simulink model "Test_07Aug2012"  (Simulink 7.7)
settings: Solver=FixedStepDiscrete  StartTime=0.0  StopTime=inf  FixedStep=0.02  RelTol=1e-3
libraries: simulink x1, utility x1
settings Model: Creator=ttcl3  LastModifiedBy=CHIEW
settings SolverCC: MaxConsecutiveMinStep=auto
settings DebuggingCC: MultiTaskRateTransMsg=warning

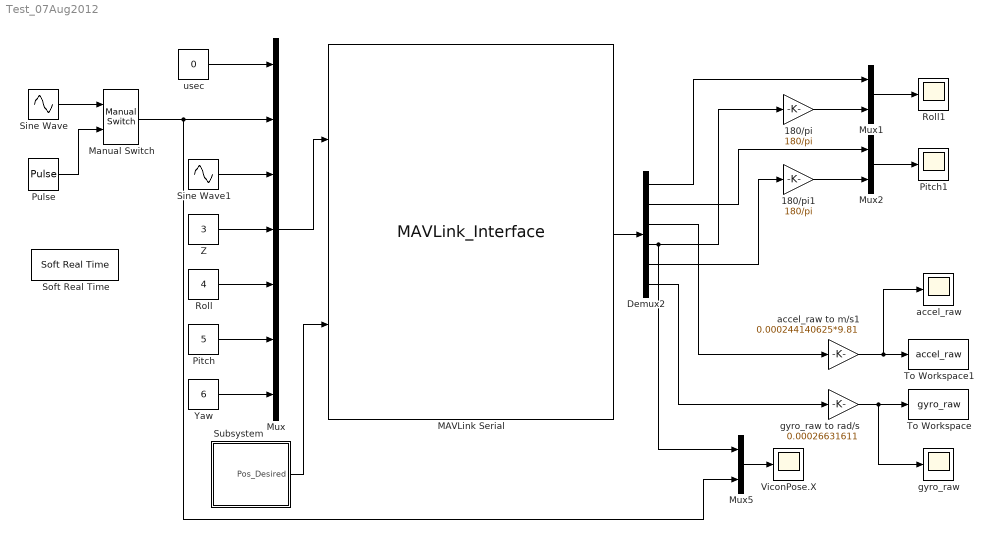
== system Test_07Aug2012 ==
  180/pi : Gain  Gain=180/pi
  180/pi1 : Gain  Gain=180/pi
  Demux2 : Demux  Outputs=6
  MAVLink Serial : S-Function  FunctionName=MAVLink_Interface  Parameters=COM_Port,Baud_Rate,MSG_INPUT,MSG_OUTPUT  EnableBusSupport=off  mask{COM_Port='COM6', Baud_Rate=57600, HEART_BEAT=off, ATTITUDE_OUT=on, RAW_IMU=off, POSITION_OUT=off, VFR_HUD=off, RC_SCALED=off, SERVO_OUT_RAW=off, VICON_XYZ_RPY_Output=off, SET_MODE=off, DATA_STREAM=off, ATTITUDE_COMMAND=off, ATTITUDE_IN=off, GPS_RAW_IN=off, VFR_HUD_IN=off, VICON_XYZ_RPY=on, VICON_VEL=off, POSITION_DESIRED=on}
      mask prompts: COM_Port "COM Port"; Baud_Rate "Baud Rate"; HEART_BEAT "HEART BEAT"; ATTITUDE_OUT "ATTITUDE"; RAW_IMU "RAW IMU"; POSITION_OUT "GLOBAL POSITION"; VFR_HUD "VFR HUD"; RC_SCALED "RC CHANNELS SCALED"; SERVO_OUT_RAW "SERVO OUTPUT RAW"; VICON_XYZ_RPY_Output "VICON Output"; SET_MODE "SET MODE"; DATA_STREAM "REQUEST DATA STREAM"; ATTITUDE_COMMAND "ATTITUDE COMMAND"; ATTITUDE_IN "ATTITUDE (HIL)"; GPS_RAW_IN "GPS RAW (HIL)"; VFR_HUD_IN "AIRSPEED (HIL)"; VICON_XYZ_RPY "VICON POSITION"; VICON_VEL "VICON SPEED"; POSITION_DESIRED "Position Desired"
      mask init:
      | MSG_ID_NUM_INPUT = [uint8(11) uint8(66) uint8(59) uint8(30) uint8(32) uint8(73) uint8(104) uint8(103) uint8(50)];
      | MSG_ID_NAME_INPUT = [SET_MODE DATA_STREAM ATTITUDE_COMMAND ATTITUDE_IN GPS_RAW_IN VFR_HUD_IN VICON_XYZ_RPY VICON_VEL POSITION_DESIRED];
      | 
      | MSG_ID_NUM_OUTPUT = [uint8(0) uint8(30) uint8(27) uint8(73) uint8(74) uint8(34) uint8(37) uint8(104)];
      | MSG_ID_NAME_OUTPUT = [HEART_BEAT ATTITUDE_OUT RAW_IMU VFR_HUD POSITION_OUT RC_SCALED SERVO_OUT_RAW VICON_XYZ_RPY_Output];
      | 
      | idx_input = find(MSG_ID_NAME_INPUT);
      | MSG_INPUT = MSG_ID_NUM_INPUT(idx_input);
      | 
      | idx_output = find(MSG_ID_NAME_OUTPUT);
      | MSG_OUTPUT = MSG_ID_NUM_OUTPUT(idx_output);
      mask TabNameString: Setting,Setting,Output Message,Output Message,Output Message,Output Message,Output Message,Output Message,Output Message,Output Message,Input Message,Input Message,Input Message,Input Message,Input Message,Input Message,Input Message,Input Message,Input Message
      mask Display:
      | %Label block
      | fprintf('MAVLink Serial\n%s\n%dbps', COM_Port,  Baud_Rate)
      | 
      | %Label input ports
      | 
      | in = 1;
      | if (SET_MODE == 1)
      |     port_label('input', in, 'SET MODE');
      |     in = in + 1;
      | end
      | if (DATA_STREAM == 1)
      |     port_label('input', in, 'REQUEST DATA STREAM');
      |     in = in + 1;
      | end
      | if (ATTITUDE_COMMAND == 1)
      |     port_label('input', in, 'ATTITUDE COMMAND');
      |     in = in + 1;
      | end
      | if (ATTITUDE_IN == 1)
      |     port_label('input', in, 'ATTITUDE (HIL)');
      |     in = in + 1;
      | end
      | if (GPS_RAW_IN == 1)
      |     port_label('input', in, 'GPS RAW (HIL)');
      |     in = in + 1;
      | end
      | if (VFR_HUD_IN == 1)
      |     port_label('input', in, 'AIRSPEED (HIL)');
      |     in = in + 1;
      | end
      | if (VICON_XYZ_RPY == 1)
      |     port_label('input', in, 'VICON XYZ RPY');
      |     in = in + 1;
      | end
      | if (VICON_VEL == 1)
      |     port_label('input', in, 'VICON_VEL');
      |     in = in + 1;
      | end
      | 
      | if (POSITION_DESIRED == 1)
      |     port_label('input', in, 'POSITION_DESIRED');
      |     in = in + 1;
      | end
      | 
      | %Label output ports
      | 
      | out = 1;
      | if (HEART_BEAT == 1)
      |     port_label('output', out, 'HEART BEAT');
      |     out = out + 1;
      | end
      | if (ATTITUDE_OUT == 1)
      |     port_label('output', out, 'ATTITUDE');
      |     out = out + 1;
      | end
      | if (RAW_IMU == 1)
      |     port_label('output', out, 'RAW IMU');
      |     out = out + 1;
      | end
      | if (POSITION_OUT == 1)
      |     port_label('output', out, 'GLOBAL POSITION');
      |     out = out + 1;
      | end
      | if (VFR_HUD == 1)
      |     port_label('output', out, 'VFR HUD');
      |     out = out + 1;
      | end
      | if (RC_SCALED == 1)
      |     port_label('output', out, 'RC CHANNELS SCALED');
      |     out = out + 1;
      | end
      | if (SERVO_OUT_RAW == 1)
      |     port_label('output', out, 'SERVO OUTPUT RAW');
      |     out = out + 1;
      | end
      | % weihua, vicon output
      | if (VICON_XYZ_RPY_Output == 1)
      |     port_label('output', out, 'VICON_XYZ_RPY');
      |     out = out + 1;
      | end
  Manual Switch : simulink/Signal Routing/Manual Switch  SystemSampleTime=-1  sw=1  action=0  varsize=off
  Mux : Mux  Inputs=7
  Mux1 : Mux  Inputs=2
  Mux2 : Mux  Inputs=2
  Mux5 : Mux  Inputs=2
  Pitch : Constant  Value=5
  Pitch1 : Scope
      settings: TickLabels=on  TimeRange=100  YMin=-35  YMax=30  SaveName=ScopeData4  SampleInput=on
  Pulse : DiscretePulseGenerator  PulseType=Time based  Period=6  PulseWidth=50  SampleTime=-1
  Roll : Constant  Value=4
  Roll1 : Scope
      settings: TickLabels=on  TimeRange=100  YMin=-35  YMax=35  SaveName=ScopeData3  SampleInput=on
  Sine Wave : Sin  Frequency=0.5  SampleTime=0.02
  Sine Wave1 : Sin  SampleTime=0.02
  Soft Real Time : utility/Soft Real Time  x=0.8
  Subsystem : Subsystem
  To Workspace : ToWorkspace  VariableName=gyro_raw  SampleTime=-1  SaveFormat=Structure With Time
  To Workspace1 : ToWorkspace  VariableName=accel_raw  SampleTime=-1  SaveFormat=Structure With Time
  ViconPose.X : Scope
      settings: TickLabels=on  TimeRange=30  YMin=-1  YMax=1  SampleInput=on
  Yaw : Constant  Value=6
  Z : Constant  Value=3
  accel_raw : Scope
      settings: TickLabels=on  TimeRange=100  YMin=-0.0275  YMax=0.0125  SampleInput=on
  accel_raw to m/s1 : Gain  Gain=0.000244140625*9.81
  gyro_raw : Scope
      settings: TickLabels=on  TimeRange=100  YMin=-0.0275  YMax=0.0125  SaveName=ScopeData2  SampleInput=on
  gyro_raw to rad/s : Gain  Gain=0.00026631611
  usec : Constant  Value=0
  wires:
  usec/1 -> Mux/1
  Sine Wave1/1 -> Mux/3
  Z/1 -> Mux/4
  Roll/1 -> Mux/5
  Pitch/1 -> Mux/6
  Yaw/1 -> Mux/7
  Mux/1 -> MAVLink Serial/1
  MAVLink Serial/1 -> Demux2/1
  Mux5/1 -> ViconPose.X/1
  Subsystem/1(Pos_Desired) -> MAVLink Serial/2
  Manual Switch/1 -> Mux/2, Mux5/2
  Sine Wave/1 -> Manual Switch/1
  Pulse/1 -> Manual Switch/2
  Demux2/1 -> Mux1/1
  Demux2/2 -> Mux2/1
  Demux2/4 -> 180/pi/1, Mux5/1
  Demux2/5 -> 180/pi1/1
  Demux2/3 -> accel_raw to m/s1/1
  accel_raw to m/s1/1 -> To Workspace1/1, accel_raw/1
  Demux2/6 -> gyro_raw to rad/s/1
  gyro_raw to rad/s/1 -> To Workspace/1, gyro_raw/1
  Mux1/1 -> Roll1/1
  Mux2/1 -> Pitch1/1
  180/pi/1 -> Mux1/2
  180/pi1/1 -> Mux2/2

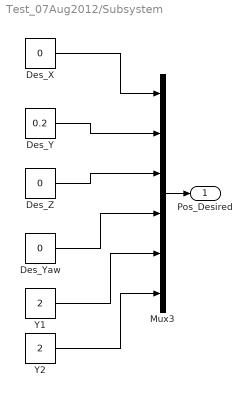
== system Test_07Aug2012/Subsystem ==
  Des_X : Constant  Value=0  SampleTime=0.02
  Des_Y : Constant  Value=0.2  SampleTime=0.02
  Des_Yaw : Constant  Value=0  SampleTime=0.02
  Des_Z : Constant  Value=0  SampleTime=0.02
  Mux3 : Mux  Inputs=6
  Y1 : Constant  Value=2  SampleTime=0.02
  Y2 : Constant  Value=2  SampleTime=0.02
  Pos_Desired : Outport
  wires:
  Des_X/1 -> Mux3/1
  Des_Y/1 -> Mux3/2
  Des_Z/1 -> Mux3/3
  Des_Yaw/1 -> Mux3/4
  Y1/1 -> Mux3/5
  Y2/1 -> Mux3/6
  Mux3/1 -> Pos_Desired/1
